simulink model "demod"  (R2016a)
settings: Solver=FixedStepDiscrete  StartTime=0.0  StopTime=inf  RelTol=1e-3
libraries: commofdm x1, dspsrcs4 x1
settings Model: Creator=senpo  LastModifiedBy=senpo

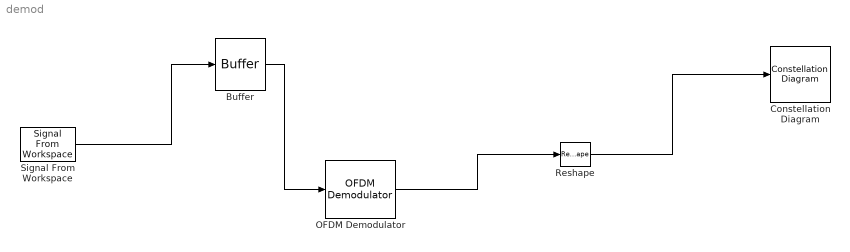
== system demod ==
  Buffer : Buffer  N=4160  TreatMby1Signals=One channel  OutputFrames=off
  Constellation Diagram : ConstellationDiagram
  OFDM Demodulator : commofdm/OFDM Demodulator  FFTLength=64  NumGuardBandCarriers=[4; 3]  RemoveDCCarrier=on  PilotOutputPort=off  PilotCarrierIndices=[12; 26; 40; 54]  CyclicPrefixLength=16  NumSymbols=52  NumReceiveAntennas=1  SimulateUsing=Interpreted execution
  Reshape : Reshape  OutputDimensions=1, []
  Signal From Workspace : dspsrcs4/Signal From Workspace  X=Signal  Ts=1e-3  nsamps=1  OutputAfterFinalValue=Cyclic repetition  ignoreOrWarnInputAndFrameLengths=off  OutputFrames=off
  wires:
  OFDM Demodulator/1 -> Reshape/1
  Reshape/1 -> Constellation Diagram/1
  Signal From Workspace/1 -> Buffer/1
  Buffer/1 -> OFDM Demodulator/1
